simulink model "mg868873"  (R2013a)
settings: Solver=FixedStepDiscrete  SolverMode=SingleTasking  StartTime=0  StopTime=10.0  FixedStep=1  RelTol=1e-3
settings Model: BufferReuse=off  Creator=djia  LastModifiedBy=hungdang
settings DataIOCC: SaveFormat=Structure  SaveState=on  OutputSaveName=yout1
settings OptimizationCC: ConditionallyExecuteInputs=off  InlineParams=on  UseFloatMulNetSlope=on  OptimizeBlockIOStorage=off  BufferReuse=off  ExpressionFolding=off  EnableMemcpy=off  PassReuseOutputArgsAs=Individual arguments  ExpressionDepthLimit=2147483647  LocalBlockOutputs=off  RollThreshold=100  DataBitsets=on  EfficientFloat2IntCast=on  EfficientMapNaN2IntZero=off  OptimizeModelRefInitCode=on  LifeSpan=1  MaxStackSize=inf  BufferReusableBoundary=off
settings DebuggingCC: WriteAfterWriteMsg=EnableAllAsError  AlgebraicLoopMsg=error  UnderspecifiedInitializationDetection=Simplified  SolverPrmCheckMsg=none  ParameterUnderflowMsg=error  ParameterPrecisionLossMsg=error  ParameterTunabilityLossMsg=error  FcnCallInpInsideContextMsg=UseLocalSettings  UnconnectedInputMsg=none  UnconnectedOutputMsg=none  ModelReferenceIOMsg=error  ModelReferenceSymbolNameMessage=none  StrictBusMsg=ErrorOnBusTreatedAsVector  NonBusSignalsTreatedAsBus=error
settings HardwareCC: ProdIntDivRoundTo=Zero  ProdEndianess=LittleEndian  ProdHWDeviceType=Atmel->AVR  TargetBitPerLong=64  TargetBitPerPointer=64  TargetIntDivRoundTo=Zero  TargetEndianess=LittleEndian  TargetWordSize=64  TargetHWDeviceType=Generic->MATLAB Host Computer
settings ModelReferenceCC: ModelReferenceNumInstancesAllowed=Zero  ModelReferencePassRootInputsByReference=off  PropagateSignalLabelsOutOfModel=on
settings RTWCC: SystemTargetFile=ert.tlc  GenCodeOnly=on  GenerateMakefile=off  TemplateMakefile=ert_default_tmf  PostCodeGenCommand=pcgscript(buildInfo)  Description=Real-Time Workshop Embedded Coder  RTWVerbose=off  RetainRTWFile=on  ProcessScript=ert_make_rtw_hook  IncludeHyperlinkInReport=on
settings CodeAppCC: ForceParamTrailComments=on  IgnoreCustomStorageClasses=off  IgnoreTestpoints=on  MaxIdLength=242  SimulinkDataObjDesc=on  SFDataObjDesc=on  MangleLength=4  CustomSymbolStrType=$N$R$M  DefineNamingRule=UpperCase  InsertBlockDesc=on  SimulinkBlockComments=off  EnableCustomComments=on  InternalIdentifier=Classic
settings ERTTargetCC: CodeReplacementLibrary=C89/C90 (ANSI)  UtilityFuncGeneration=Shared location  ERTMultiwordTypeDef=User defined  ERTMultiwordLength=711  IncludeMdlTerminateFcn=off  GeneratePreprocessorConditionals=Disable all  CombineOutputUpdateFcns=off  SuppressErrorStatus=on  IncludeFileDelimiter=UseQuote  SupportAbsoluteTime=off  SupportNonFinite=off  ParenthesesLevel=Maximum  MultiInstanceErrorCode=None  ERTCustomFileTemplate=example_file_process.tlc  SignalDisplayLevel=1  ParamTuneLevel=6  ERTFilePackagingFormat=CompactWithDataFile  PreserveIfCondition=on  SuppressUnreachableDefaultCases=on

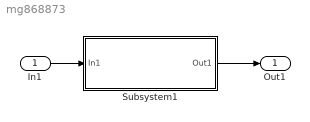
== system mg868873 ==
  In1 : Inport  PortDimensions=10
  Subsystem1 : Subsystem  TreatAsAtomicUnit=on
      settings: RTWFileNameOpts=Use function name
  Out1 : Outport
  wires:
  In1/1 -> Subsystem1/1(In1)
  Subsystem1/1(Out1) -> Out1/1

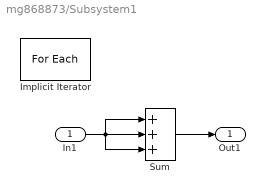
== system mg868873/Subsystem1 ==
  In1 : Inport  Partition=on  PartitionDimension=1  PartitionWidth=1
  Implicit Iterator : ForEach  IndexMode=One-based  StateHandling=Same state for all iterations  StateReset=reset
  Sum : Sum  Inputs=3
  Out1 : Outport  ConcatenationDimension=1
  wires:
  Sum/1 -> Out1/1
  In1/1 -> Sum/2, Sum/1, Sum/3
